simulink model "SWC_FDC_type"  (R2021b)
settings: Solver=FixedStepDiscrete  StartTime=0.0  StopTime=10.0  FixedStep=0.001  RelTol=1e-3
values from neighbouring files (symbols this model uses):
  C_TASK_5MS_S = (	C_TICK_TIME_S      	)    [vcu_local_hdr.m]
  DID_VCUKey = uint16(0x0202)    [vcu_local_hdr.m]
  DID_XWD = uint16(513)    [vcu_local_hdr.m]
  DIDLen_DKCKey = uint16(8)    [vcu_local_hdr.m]
  DIDLen_FoxPiBattSta = uint16(4)    [vcu_local_hdr.m]
  DIDLen_FoxPiBrakeSta = uint16(13)    [vcu_local_hdr.m]
  DIDLen_FoxPiButtonSta = uint16(2)    [vcu_local_hdr.m]
  DIDLen_FoxPiCtrlEnSw = uint16(1)    [vcu_local_hdr.m]
  DIDLen_FoxPiDrivingCtrl = uint16(21)    [vcu_local_hdr.m]
  DIDLen_FoxPiEPSSta = uint16(11)    [vcu_local_hdr.m]
  DIDLen_FoxPiLampCtrl = uint16(6)    [vcu_local_hdr.m]
  DIDLen_FoxPiLampSta = uint16(2)    [vcu_local_hdr.m]
  DIDLen_FoxPiMotionSta = uint16(13)    [vcu_local_hdr.m]
  DIDLen_FoxPiMotorSta = uint16(11)    [vcu_local_hdr.m]
  DIDLen_FoxPiPedalPos = uint16(3)    [vcu_local_hdr.m]
  DIDLen_FoxPiPTGUSSSw = uint16(1)    [vcu_local_hdr.m]
  DIDLen_FoxPiShifterAllow = uint16(3)    [vcu_local_hdr.m]
  DIDLen_FoxPiSwSta = uint16(2)    [vcu_local_hdr.m]
  DIDLen_FoxPiTPMSSta = uint16(13)    [vcu_local_hdr.m]
  DIDLen_FoxPiUSSDist = uint16(20)    [vcu_local_hdr.m]
  DIDLen_FoxPiUSSFaultSta = uint16(2)    [vcu_local_hdr.m]
  DIDLen_FoxPiWheelSpd = uint16(16)    [vcu_local_hdr.m]
  DIDNum_DKCKey = uint16(0x0202)    [vcu_local_hdr.m]
  DIDNum_FoxPiBattSta = uint16(0x100D)    [vcu_local_hdr.m]
  DIDNum_FoxPiBrakeSta = uint16(0x1003)    [vcu_local_hdr.m]
  DIDNum_FoxPiButtonSta = uint16(0x1006)    [vcu_local_hdr.m]
  DIDNum_FoxPiCtrlEnSw = uint16(0x1012)    [vcu_local_hdr.m]
  DIDNum_FoxPiDrivingCtrl = uint16(0x1001)    [vcu_local_hdr.m]
  DIDNum_FoxPiEPSSta = uint16(0x1005)    [vcu_local_hdr.m]
  DIDNum_FoxPiLampCtrl = uint16(0x100C)    [vcu_local_hdr.m]
  DIDNum_FoxPiLampSta = uint16(0x100B)    [vcu_local_hdr.m]
  DIDNum_FoxPiMotionSta = uint16(0x1002)    [vcu_local_hdr.m]
  DIDNum_FoxPiMotorSta = uint16(0x1010)    [vcu_local_hdr.m]
  DIDNum_FoxPiPedalPos = uint16(0x100F)    [vcu_local_hdr.m]
  DIDNum_FoxPiPTGUSSSw = uint16(0x1009)    [vcu_local_hdr.m]
  DIDNum_FoxPiShifterAllow = uint16(0x1011)    [vcu_local_hdr.m]
  DIDNum_FoxPiSwSta = uint16(0x100A)    [vcu_local_hdr.m]
  DIDNum_FoxPiTPMSSta = uint16(0x100E)    [vcu_local_hdr.m]
  DIDNum_FoxPiUSSDist = uint16(0x1007)    [vcu_local_hdr.m]
  DIDNum_FoxPiUSSFaultSta = uint16(0x1008)    [vcu_local_hdr.m]
  DIDNum_FoxPiWheelSpd = uint16(0x1004)    [vcu_local_hdr.m]
  DIDVCUKeyLength = uint16(8)    [vcu_local_hdr.m]
  DTC_10020B = Simulink.Parameter    [DTC_Constant_Definition.m]
  DTC_10020C = Simulink.Parameter    [DTC_Constant_Definition.m]
  DTC_10020D = Simulink.Parameter    [DTC_Constant_Definition.m]
  DTC_10020E = Simulink.Parameter    [DTC_Constant_Definition.m]
  DTC_100210 = Simulink.Parameter    [DTC_Constant_Definition.m]
  DTC_100211 = Simulink.Parameter    [DTC_Constant_Definition.m]
  DTC_100212 = Simulink.Parameter    [DTC_Constant_Definition.m]
  DTC_100213 = Simulink.Parameter    [DTC_Constant_Definition.m]
  DTC_100214 = Simulink.Parameter    [DTC_Constant_Definition.m]
  DTC_100215 = Simulink.Parameter    [DTC_Constant_Definition.m]
  DTC_100216 = Simulink.Parameter    [DTC_Constant_Definition.m]
  DTC_100217 = Simulink.Parameter    [DTC_Constant_Definition.m]
  DTC_100218 = Simulink.Parameter    [DTC_Constant_Definition.m]
  DTC_100219 = Simulink.Parameter    [DTC_Constant_Definition.m]
  DTC_10021A = Simulink.Parameter    [DTC_Constant_Definition.m]
  DTC_10021B = Simulink.Parameter    [DTC_Constant_Definition.m]
  DTC_10021C = Simulink.Parameter    [DTC_Constant_Definition.m]
  DTC_10021D = Simulink.Parameter    [DTC_Constant_Definition.m]
  DTC_10021E = Simulink.Parameter    [DTC_Constant_Definition.m]
  DTC_100220 = Simulink.Parameter    [DTC_Constant_Definition.m]
  DTC_100221 = Simulink.Parameter    [DTC_Constant_Definition.m]
  DTC_100223 = Simulink.Parameter    [DTC_Constant_Definition.m]
  DTC_100224 = Simulink.Parameter    [DTC_Constant_Definition.m]
  DTC_100225 = Simulink.Parameter    [DTC_Constant_Definition.m]
  DTC_100226 = Simulink.Parameter    [DTC_Constant_Definition.m]
  DTC_100227 = Simulink.Parameter    [DTC_Constant_Definition.m]
  DTC_100242 = Simulink.Parameter    [DTC_Constant_Definition.m]
  DTC_100243 = Simulink.Parameter    [DTC_Constant_Definition.m]
  DTC_100244 = Simulink.Parameter    [DTC_Constant_Definition.m]
  DTC_100247 = Simulink.Parameter    [DTC_Constant_Definition.m]
  DTC_100248 = Simulink.Parameter    [DTC_Constant_Definition.m]
  DTC_100249 = Simulink.Parameter    [DTC_Constant_Definition.m]
  DTC_100250 = Simulink.Parameter    [DTC_Constant_Definition.m]
  DTC_100251 = Simulink.Parameter    [DTC_Constant_Definition.m]
  DTC_100252 = Simulink.Parameter    [DTC_Constant_Definition.m]
  DTC_100A10 = Simulink.Parameter    [DTC_Constant_Definition.m]
  DTC_100A12 = Simulink.Parameter    [DTC_Constant_Definition.m]
  DTC_100A16 = Simulink.Parameter    [DTC_Constant_Definition.m]
  DTC_100A17 = Simulink.Parameter    [DTC_Constant_Definition.m]
  DTC_100A18 = Simulink.Parameter    [DTC_Constant_Definition.m]
  DTC_100A19 = Simulink.Parameter    [DTC_Constant_Definition.m]
  DTC_500B01 = Simulink.Parameter    [DTC_Constant_Definition.m]
  DTC_500B02 = Simulink.Parameter    [DTC_Constant_Definition.m]
  DTC_500B03 = Simulink.Parameter    [DTC_Constant_Definition.m]
  DTC_500B04 = Simulink.Parameter    [DTC_Constant_Definition.m]
  DTC_500B05 = Simulink.Parameter    [DTC_Constant_Definition.m]
  DTC_500B06 = Simulink.Parameter    [DTC_Constant_Definition.m]
  DTC_500B07 = Simulink.Parameter    [DTC_Constant_Definition.m]
  DTC_500B08 = Simulink.Parameter    [DTC_Constant_Definition.m]
  DTC_500B09 = Simulink.Parameter    [DTC_Constant_Definition.m]
  DTC_500B0A = Simulink.Parameter    [DTC_Constant_Definition.m]
  DTC_500B0B = Simulink.Parameter    [DTC_Constant_Definition.m]
  DTC_500B0C = Simulink.Parameter    [DTC_Constant_Definition.m]
  DTC_500B0D = Simulink.Parameter    [DTC_Constant_Definition.m]
  DTC_500B0E = Simulink.Parameter    [DTC_Constant_Definition.m]
  DTC_500B0F = Simulink.Parameter    [DTC_Constant_Definition.m]
  DTC_500B10 = Simulink.Parameter    [DTC_Constant_Definition.m]
  DTC_90021F = Simulink.Parameter    [DTC_Constant_Definition.m]
  DTC_90022F = Simulink.Parameter    [DTC_Constant_Definition.m]
  DTC_900253 = Simulink.Parameter    [DTC_Constant_Definition.m]
  DTC_900254 = Simulink.Parameter    [DTC_Constant_Definition.m]
  DTC_900301 = Simulink.Parameter    [DTC_Constant_Definition.m]
  DTC_900302 = Simulink.Parameter    [DTC_Constant_Definition.m]
  DTC_900303 = Simulink.Parameter    [DTC_Constant_Definition.m]
  DTC_900304 = Simulink.Parameter    [DTC_Constant_Definition.m]
  DTC_900305 = Simulink.Parameter    [DTC_Constant_Definition.m]
  DTC_900909 = Simulink.Parameter    [DTC_Constant_Definition.m]
  DTC_90090A = Simulink.Parameter    [DTC_Constant_Definition.m]
  DTC_90090B = Simulink.Parameter    [DTC_Constant_Definition.m]
  DTC_90090C = Simulink.Parameter    [DTC_Constant_Definition.m]
  DTC_90090D = Simulink.Parameter    [DTC_Constant_Definition.m]
  DTC_90090E = Simulink.Parameter    [DTC_Constant_Definition.m]
  DTC_90090F = Simulink.Parameter    [DTC_Constant_Definition.m]
  DTC_900910 = Simulink.Parameter    [DTC_Constant_Definition.m]
  DTC_900911 = Simulink.Parameter    [DTC_Constant_Definition.m]
  DTC_900912 = Simulink.Parameter    [DTC_Constant_Definition.m]
  DTC_900913 = Simulink.Parameter    [DTC_Constant_Definition.m]
  DTC_900914 = Simulink.Parameter    [DTC_Constant_Definition.m]
  ... (+54 more)
undefined symbols (not defined in the file or in its folder): f32_ApsOutVehSpdSig, KHAL_CANBusOffDebounce_cnt, KHAL_CANBusOffDebounce_s, KHAL_DKCDecryptEnable_flg_ovrdflg, KHAL_DKCDecryptEnable_flg_ovrdval, KHAL_RandomNumberY1_enum, KHAL_RandomNumberY2_enum, KHAL_RandomNumberY_ovrdflg, KHAL_TPMSRESBUTT_flg_ovrdflg, KHAL_TPMSRESBUTT_flg_ovrdval, KINP_ReadVinCode_flg, P_boolean, R_DIDWriteCDD_CSOP_DIDSet_DKCKey, R_DIDWriteCDD_CSOP_DIDSet_FoxPiBattSta, R_DIDWriteCDD_CSOP_DIDSet_FoxPiBrakeSta, R_DIDWriteCDD_CSOP_DIDSet_FoxPiButtonSta, R_DIDWriteCDD_CSOP_DIDSet_FoxPiCtrlEnSw, R_DIDWriteCDD_CSOP_DIDSet_FoxPiDrivingCtrl, R_DIDWriteCDD_CSOP_DIDSet_FoxPiEPSSta, R_DIDWriteCDD_CSOP_DIDSet_FoxPiLampCtrl, R_DIDWriteCDD_CSOP_DIDSet_FoxPiLampSta, R_DIDWriteCDD_CSOP_DIDSet_FoxPiMotionSta, R_DIDWriteCDD_CSOP_DIDSet_FoxPiMotorSta, R_DIDWriteCDD_CSOP_DIDSet_FoxPiPedalPos, R_DIDWriteCDD_CSOP_DIDSet_FoxPiPTGUSSSw, R_DIDWriteCDD_CSOP_DIDSet_FoxPiShifterAllow, R_DIDWriteCDD_CSOP_DIDSet_FoxPiSwSta, R_DIDWriteCDD_CSOP_DIDSet_FoxPiTPMSSta, R_DIDWriteCDD_CSOP_DIDSet_FoxPiUSSDist, R_DIDWriteCDD_CSOP_DIDSet_FoxPiUSSFaultSta, R_DIDWriteCDD_CSOP_DIDSet_FoxPiWheelSpd, R_E2E_CAN3_VCU1_CSOP_Write_CAN3_VCU1, R_E2E_CAN3_VCU1_toNIDEC_CSOP_Write_CAN3_VCU1_toNIDEC, R_E2E_CAN4_VCU1_CSOP_Write_CAN4_VCU1, R_FDCCDD_Inner_CSOP_FDC_AppCallSleep, R_HALIN_IMU_CSOP_IMUSetSta, R_HALINCDD_CSOP_PAS_Handler, R_HALINCDD_CSOP_ResetPedalZeroPosDone, R_HALINCDD_CSOP_TPMSSensorIDRegSetResults, R_HALINCDD_CSOP_UDS_Main, R_HALOUT_APS_CSOP_ApsOutput, R_HALOUTCDD_CSOP_AppNmStateReq, R_HALOUTCDD_CSOP_IVIReset, R_HALOUTCDD_CSOP_SetAcoreRebootCmdACK, R_HALOUTCDD_CSOP_SetSysPwrStat ... (+80)
libraries: FVT_lib x447, simulink x289, hcu_lib x19, hdlsllib x9, app x1, halin x1, halout x1, matrix_library x1, inp x1, outp x1
(part 13 of 15)

== system SWC_FDC_type/run_SWC_FDC_RxTx_5ms_sys/Halin_CDD/Halin_TPMS/Subsystem ==
  note: Custom State Judgement
  note: Data Output
  note: Data Valid Judge
  TPMS_DataIn_flg : Inport
  TPMS_RawData : Inport  Port=2
  Add : Sum  Inputs=++++
  Bit Shift : hdlsllib/Logic and Bit Operations/Bit Shift  mode=Shift Left Logical  N=24
  Bit Shift1 : hdlsllib/Logic and Bit Operations/Bit Shift  mode=Shift Left Logical  N=16
  Bit Shift3 : hdlsllib/Logic and Bit Operations/Bit Shift  mode=Shift Left Logical  N=8
  Bitwise NOT : simulink/Logic and Bit Operations/Bitwise Operator  logicop=NOT  UseBitMask=off  BitMask=bin2dec('11011001')  BitMaskRealWorld=Stored Integer
  CRC8_Caculation : Subsystem
  Constant1 : Constant  Value=ENUM_TPMSSTA_TRIGGER
  Constant{4,7,9..10} (4 alike) : Constant  Value=TRUE
  Constant{5..6,8,11} (4 alike) : Constant  Value=FALSE
  Constant2 : Constant  Value=ENUM_TPMSSTA_LOWBATTERY
  Constant3 : Constant  Value=ENUM_TPMSSTA_FAT
  Data Type Conversion : DataTypeConversion  OutDataTypeStr=uint32
  Data Type Conversion1 : DataTypeConversion  OutDataTypeStr=uint8
  Data Type Conversion2 : DataTypeConversion  OutDataTypeStr=uint8
  Data Type Conversion3 : DataTypeConversion  OutDataTypeStr=uint32
  Data Type Conversion4 : DataTypeConversion  OutDataTypeStr=uint32
  Demux : Demux  Outputs=9
  Demux1 : Demux  Outputs=10
  Equal{,1..4} (5 alike) : RelationalOperator  Operator===  OutDataTypeStr=boolean  RndMeth=Simplest
  Logical Operator : Logic  Inputs=3  AllPortsSameDT=off  OutDataTypeStr=boolean
  Mux : Mux  Inputs=10
  Mux1 : Mux  Inputs=8
  Switch{,1..4} (5 alike) : Switch  Criteria=u2 ~= 0
  Unit Delay : UnitDelay  SampleTime=-1  HasFrameUpgradeWarning=on
  VHAL_TPMSDataIn_flg : Outport
  VHAL_TPMSID_raw : Outport  Port=2
  VHAL_TPMSPressure_raw : Outport  Port=3
  VHAL_TPMSTemp_raw : Outport  Port=4
  VHAL_TPMSSta_enum : Outport  Port=5
  VHAL_TPMSPressureMi_raw : Outport  Port=6
  VHAL_TPMSCRC_crc : Outport  Port=7
  VHAL_TPMSCRCCalc_crc : Outport  Port=8
  VHAL_TPMSFAT_flg : Outport  Port=9
  VHAL_TPMSBattLow_flg : Outport  Port=10
  VHAL_TPMSTrigger_flg : Outport  Port=11
  wires:
  TPMS_DataIn_flg/1 -> Data Type Conversion2/1
  [TPMSData] -> Demux/1
  Bit Shift/1 -> Add/1
  Bit Shift1/1 -> Add/2
  Bit Shift3/1 -> Add/3
  Add/1 -> VHAL_TPMSID_raw/1
  Demux/5 -> [Pressure]  "Pressure"
  Demux/7 -> [Status]  "Sta"
  Demux/8 -> [PressureMirror]  "PressureMirror"
  Demux/9 -> [CRC]  "CRC"
  Demux/1 -> [ID4]  "ID4"
  Demux/2 -> [ID3]  "ID3"
  Demux/3 -> [ID2]  "ID2"
  Demux/4 -> [ID1]  "ID1"
  Demux/6 -> [Temp]  "Temp"
  [Pressure] -> Bitwise NOT/1
  Bitwise NOT/1 -> Equal/1
  [PressureMirror] -> Equal/2
  [ID4] -> Mux1/1
  [ID3] -> Mux1/2
  [ID2] -> Mux1/3
  [ID1] -> Mux1/4
  [Pressure] -> Mux1/5
  [Temp] -> Mux1/6
  [Status] -> Mux1/7
  [PressureMirror] -> Mux1/8
  Mux1/1 -> CRC8_Caculation/1(MsgData)
  [CRC] -> Equal1/2
  Equal1/1 -> Logical Operator/1
  Equal/1 -> Logical Operator/2
  Logical Operator/1 -> [DataValid_flg]
  [DataValid_flg] -> Switch/2
  Mux/1 -> Switch/1
  Switch/1 -> Unit Delay/1, Demux1/1
  Unit Delay/1 -> Switch/3
  Data Type Conversion1/1 -> [TPMSData]
  Data Type Conversion2/1 -> [Data_in]
  CRC8_Caculation/1(CRCout) -> [CRC_Calc], Equal1/1  "CRC_Calc"
  Switch1/1 -> VHAL_TPMSFAT_flg/1
  [VHAL_TPMSSta_enum] -> Equal2/1
  Constant3/1 -> Equal2/2
  Equal2/1 -> Switch1/2
  Constant4/1 -> Switch1/1
  Constant5/1 -> Switch1/3
  Constant8/1 -> Switch2/3
  [VHAL_TPMSSta_enum] -> Equal3/1
  Constant7/1 -> Switch2/1
  Switch2/1 -> VHAL_TPMSBattLow_flg/1
  Equal3/1 -> Switch2/2
  Constant2/1 -> Equal3/2
  [Data_in] -> Logical Operator/3
  [DataValid_flg] -> Switch3/2
  Switch3/1 -> VHAL_TPMSDataIn_flg/1
  Constant6/1 -> Switch3/3
  Constant9/1 -> Switch3/1
  [ID4] -> Mux/1
  [ID3] -> Mux/2
  [ID2] -> Mux/3
  [ID1] -> Mux/4
  [Pressure] -> Mux/5
  [Temp] -> Mux/6
  [Status] -> Mux/7
  [PressureMirror] -> Mux/8
  [CRC] -> Mux/9
  [CRC_Calc] -> Mux/10
  Demux1/10 -> VHAL_TPMSCRCCalc_crc/1
  Demux1/9 -> VHAL_TPMSCRC_crc/1
  Demux1/8 -> VHAL_TPMSPressureMi_raw/1
  Demux1/7 -> [VHAL_TPMSSta_enum], VHAL_TPMSSta_enum/1
  Demux1/6 -> VHAL_TPMSTemp_raw/1
  Demux1/5 -> VHAL_TPMSPressure_raw/1
  Demux1/1 -> Data Type Conversion/1
  Demux1/2 -> Data Type Conversion3/1
  Demux1/3 -> Data Type Conversion4/1
  Data Type Conversion/1 -> Bit Shift/1
  Data Type Conversion3/1 -> Bit Shift1/1
  Data Type Conversion4/1 -> Bit Shift3/1
  Demux1/4 -> Add/4
  TPMS_RawData/1 -> Data Type Conversion1/1
  [VHAL_TPMSSta_enum] -> Equal4/1
  Constant1/1 -> Equal4/2
  Equal4/1 -> Switch4/2
  Constant10/1 -> Switch4/1
  Constant11/1 -> Switch4/3
  Switch4/1 -> VHAL_TPMSTrigger_flg/1

== system SWC_FDC_type/run_SWC_FDC_RxTx_5ms_sys/OUTP_AFTER/DID_list/pct2raw1 ==
  EAPS1_pct : Inport
  EAPS2_pct : Inport  Port=2
  Bitwise AND1 : simulink/Logic and Bit Operations/Bitwise Operator  logicop=AND  UseBitMask=on  BitMask=0xF  BitMaskRealWorld=Stored Integer
  Bitwise AND2 : simulink/Logic and Bit Operations/Bitwise Operator  logicop=AND  UseBitMask=on  BitMask=0xFF0  BitMaskRealWorld=Stored Integer
  Bitwise AND3 : simulink/Logic and Bit Operations/Bitwise Operator  logicop=AND  UseBitMask=on  BitMask=0xFF  BitMaskRealWorld=Stored Integer
  Bitwise AND4 : simulink/Logic and Bit Operations/Bitwise Operator  logicop=AND  UseBitMask=on  BitMask=0xF00  BitMaskRealWorld=Stored Integer
  Bitwise AND5 : simulink/Logic and Bit Operations/Bitwise Operator  logicop=OR  UseBitMask=off  NumInputPorts=2  BitMask=0xFF  BitMaskRealWorld=Stored Integer
  Data Type Conversion1 : DataTypeConversion  OutDataTypeStr=uint8
  Data Type Conversion2 : DataTypeConversion  OutDataTypeStr=uint16
  Data Type Conversion3 : DataTypeConversion  OutDataTypeStr=uint8
  Data Type Conversion4 : DataTypeConversion  OutDataTypeStr=uint16
  Data Type Conversion5 : DataTypeConversion  OutDataTypeStr=uint8
  Gain : Gain  Gain=1/20
  Gain1 : Gain  Gain=1/40
  Mux2 : Mux  Inputs=3
  Shift Arithmetic1 : ArithShift  BitShiftNumber=8  BitShiftDirection=Right
  Shift Arithmetic2 : ArithShift  BitShiftNumber=4  BitShiftDirection=Left
  Shift Arithmetic39 : ArithShift  BitShiftNumber=4  BitShiftDirection=Right
  convert_out1 : FVT_lib/hal/convert_out  gain=0.001  offset=0
  convert_out4 : FVT_lib/hal/convert_out  gain=0.001  offset=0
  PedalZP_raw8 : Outport
  wires:
  Data Type Conversion1/1 -> Mux2/2
  Bitwise AND5/1 -> Data Type Conversion1/1
  Shift Arithmetic1/1 -> Bitwise AND5/2
  Shift Arithmetic2/1 -> Bitwise AND5/1
  Gain1/1 -> convert_out1/1
  Gain/1 -> convert_out4/1
  EAPS1_pct/1 -> Gain/1
  convert_out4/1 -> Data Type Conversion2/1
  convert_out1/1 -> Data Type Conversion4/1
  EAPS2_pct/1 -> Gain1/1
  Bitwise AND3/1 -> Data Type Conversion3/1
  Bitwise AND4/1 -> Shift Arithmetic1/1
  Data Type Conversion4/1 -> Bitwise AND3/1, Bitwise AND4/1
  Data Type Conversion3/1 -> Mux2/3
  Data Type Conversion5/1 -> Mux2/1
  Data Type Conversion2/1 -> Bitwise AND2/1, Bitwise AND1/1
  Bitwise AND2/1 -> Shift Arithmetic39/1
  Shift Arithmetic39/1 -> Data Type Conversion5/1
  Mux2/1 -> PedalZP_raw8/1
  Bitwise AND1/1 -> Shift Arithmetic2/1

== system SWC_FDC_type/run_SWC_FDC_RxTx_5ms_sys/OUTP_AFTER/DID_list/pct2raw8 ==
  EAPS1_pct : Inport
  EAPS2_pct : Inport  Port=2
  Bitwise AND1 : simulink/Logic and Bit Operations/Bitwise Operator  logicop=AND  UseBitMask=on  BitMask=0xF  BitMaskRealWorld=Stored Integer
  Bitwise AND2 : simulink/Logic and Bit Operations/Bitwise Operator  logicop=AND  UseBitMask=on  BitMask=0xFF0  BitMaskRealWorld=Stored Integer
  Bitwise AND3 : simulink/Logic and Bit Operations/Bitwise Operator  logicop=AND  UseBitMask=on  BitMask=0xFF  BitMaskRealWorld=Stored Integer
  Bitwise AND4 : simulink/Logic and Bit Operations/Bitwise Operator  logicop=AND  UseBitMask=on  BitMask=0xF00  BitMaskRealWorld=Stored Integer
  Bitwise AND5 : simulink/Logic and Bit Operations/Bitwise Operator  logicop=OR  UseBitMask=off  NumInputPorts=2  BitMask=0xFF  BitMaskRealWorld=Stored Integer
  Data Type Conversion1 : DataTypeConversion  OutDataTypeStr=uint8
  Data Type Conversion2 : DataTypeConversion  OutDataTypeStr=uint16
  Data Type Conversion3 : DataTypeConversion  OutDataTypeStr=uint8
  Data Type Conversion4 : DataTypeConversion  OutDataTypeStr=uint16
  Data Type Conversion5 : DataTypeConversion  OutDataTypeStr=uint8
  Gain : Gain  Gain=1/20
  Gain1 : Gain  Gain=1/40
  Mux2 : Mux  Inputs=3
  Shift Arithmetic1 : ArithShift  BitShiftNumber=8  BitShiftDirection=Right
  Shift Arithmetic2 : ArithShift  BitShiftNumber=4  BitShiftDirection=Left
  Shift Arithmetic39 : ArithShift  BitShiftNumber=4  BitShiftDirection=Right
  convert_out1 : FVT_lib/hal/convert_out  gain=0.001  offset=0
  convert_out4 : FVT_lib/hal/convert_out  gain=0.001  offset=0
  PedalZP_raw8 : Outport
  wires:
  Bitwise AND1/1 -> Shift Arithmetic2/1
  Mux2/1 -> PedalZP_raw8/1
  Shift Arithmetic39/1 -> Data Type Conversion5/1
  Bitwise AND2/1 -> Shift Arithmetic39/1
  Data Type Conversion2/1 -> Bitwise AND1/1, Bitwise AND2/1
  Data Type Conversion5/1 -> Mux2/1
  Data Type Conversion3/1 -> Mux2/3
  Data Type Conversion4/1 -> Bitwise AND4/1, Bitwise AND3/1
  Bitwise AND4/1 -> Shift Arithmetic1/1
  Bitwise AND3/1 -> Data Type Conversion3/1
  EAPS2_pct/1 -> Gain1/1
  convert_out1/1 -> Data Type Conversion4/1
  convert_out4/1 -> Data Type Conversion2/1
  EAPS1_pct/1 -> Gain/1
  Gain/1 -> convert_out4/1
  Gain1/1 -> convert_out1/1
  Shift Arithmetic2/1 -> Bitwise AND5/1
  Shift Arithmetic1/1 -> Bitwise AND5/2
  Bitwise AND5/1 -> Data Type Conversion1/1
  Data Type Conversion1/1 -> Mux2/2

== system SWC_FDC_type/run_SWC_FDC_RxTx_5ms_sys/OUTP_AFTER/DID_list/uint32Touint8Array ==
  In1 : Inport
  Bitwise AND1 : simulink/Logic and Bit Operations/Bitwise Operator  logicop=AND  UseBitMask=on  BitMask=bin2dec('00000000000000000000000011111111')  BitMaskRealWorld=Stored Integer
  Bitwise AND2 : simulink/Logic and Bit Operations/Bitwise Operator  logicop=AND  UseBitMask=on  BitMask=bin2dec('00000000000000001111111100000000')  BitMaskRealWorld=Stored Integer
  Bitwise AND3 : simulink/Logic and Bit Operations/Bitwise Operator  logicop=AND  UseBitMask=on  BitMask=bin2dec('00000000111111110000000000000000')  BitMaskRealWorld=Stored Integer
  Bitwise AND4 : simulink/Logic and Bit Operations/Bitwise Operator  logicop=AND  UseBitMask=on  BitMask=bin2dec('11111111000000000000000000000000')  BitMaskRealWorld=Stored Integer
  Data Type Conversion{1,3..5} (4 alike) : DataTypeConversion  OutDataTypeStr=uint8
  Data Type Conversion2 : DataTypeConversion  OutDataTypeStr=uint32
  Mux2 : Mux
  Shift Arithmetic39 : ArithShift  BitShiftNumber=8  BitShiftDirection=Right
  Shift Arithmetic40 : ArithShift  BitShiftNumber=16  BitShiftDirection=Right
  Shift Arithmetic41 : ArithShift  BitShiftNumber=24  BitShiftDirection=Right
  Out1 : Outport
  wires:
  Bitwise AND4/1 -> Shift Arithmetic41/1
  Bitwise AND1/1 -> Data Type Conversion1/1
  Shift Arithmetic40/1 -> Data Type Conversion4/1
  Shift Arithmetic41/1 -> Data Type Conversion3/1
  Mux2/1 -> Out1/1
  In1/1 -> Data Type Conversion2/1
  Bitwise AND3/1 -> Shift Arithmetic40/1
  Shift Arithmetic39/1 -> Data Type Conversion5/1
  Data Type Conversion3/1 -> Mux2/1
  Bitwise AND2/1 -> Shift Arithmetic39/1
  Data Type Conversion2/1 -> Bitwise AND4/1, Bitwise AND3/1, Bitwise AND1/1, Bitwise AND2/1
  Data Type Conversion5/1 -> Mux2/3
  Data Type Conversion4/1 -> Mux2/2
  Data Type Conversion1/1 -> Mux2/4

== system SWC_FDC_type/run_SWC_FDC_RxTx_5ms_sys/OUTP_AFTER/DID_list/uint32Touint8Array1 ==
  In1 : Inport
  Bitwise AND1 : simulink/Logic and Bit Operations/Bitwise Operator  logicop=AND  UseBitMask=on  BitMask=bin2dec('00000000000000000000000011111111')  BitMaskRealWorld=Stored Integer
  Bitwise AND2 : simulink/Logic and Bit Operations/Bitwise Operator  logicop=AND  UseBitMask=on  BitMask=bin2dec('00000000000000001111111100000000')  BitMaskRealWorld=Stored Integer
  Bitwise AND3 : simulink/Logic and Bit Operations/Bitwise Operator  logicop=AND  UseBitMask=on  BitMask=bin2dec('00000000111111110000000000000000')  BitMaskRealWorld=Stored Integer
  Bitwise AND4 : simulink/Logic and Bit Operations/Bitwise Operator  logicop=AND  UseBitMask=on  BitMask=bin2dec('11111111000000000000000000000000')  BitMaskRealWorld=Stored Integer
  Data Type Conversion{1,3..5} (4 alike) : DataTypeConversion  OutDataTypeStr=uint8
  Data Type Conversion2 : DataTypeConversion  OutDataTypeStr=uint32
  Mux2 : Mux
  Shift Arithmetic39 : ArithShift  BitShiftNumber=8  BitShiftDirection=Right
  Shift Arithmetic40 : ArithShift  BitShiftNumber=16  BitShiftDirection=Right
  Shift Arithmetic41 : ArithShift  BitShiftNumber=24  BitShiftDirection=Right
  Out1 : Outport
  wires:
  Data Type Conversion1/1 -> Mux2/4
  Data Type Conversion4/1 -> Mux2/2
  Data Type Conversion5/1 -> Mux2/3
  Data Type Conversion2/1 -> Bitwise AND2/1, Bitwise AND1/1, Bitwise AND3/1, Bitwise AND4/1
  Bitwise AND2/1 -> Shift Arithmetic39/1
  Data Type Conversion3/1 -> Mux2/1
  Shift Arithmetic39/1 -> Data Type Conversion5/1
  Bitwise AND3/1 -> Shift Arithmetic40/1
  In1/1 -> Data Type Conversion2/1
  Mux2/1 -> Out1/1
  Shift Arithmetic41/1 -> Data Type Conversion3/1
  Shift Arithmetic40/1 -> Data Type Conversion4/1
  Bitwise AND1/1 -> Data Type Conversion1/1
  Bitwise AND4/1 -> Shift Arithmetic41/1

== system SWC_FDC_type/run_SWC_FDC_RxTx_5ms_sys/OUTP_AFTER/DID_list/uint32Touint8Array2 ==
  In1 : Inport
  Bitwise AND1 : simulink/Logic and Bit Operations/Bitwise Operator  logicop=AND  UseBitMask=on  BitMask=bin2dec('00000000000000000000000011111111')  BitMaskRealWorld=Stored Integer
  Bitwise AND2 : simulink/Logic and Bit Operations/Bitwise Operator  logicop=AND  UseBitMask=on  BitMask=bin2dec('00000000000000001111111100000000')  BitMaskRealWorld=Stored Integer
  Bitwise AND3 : simulink/Logic and Bit Operations/Bitwise Operator  logicop=AND  UseBitMask=on  BitMask=bin2dec('00000000111111110000000000000000')  BitMaskRealWorld=Stored Integer
  Bitwise AND4 : simulink/Logic and Bit Operations/Bitwise Operator  logicop=AND  UseBitMask=on  BitMask=bin2dec('11111111000000000000000000000000')  BitMaskRealWorld=Stored Integer
  Data Type Conversion{1,3..5} (4 alike) : DataTypeConversion  OutDataTypeStr=uint8
  Data Type Conversion2 : DataTypeConversion  OutDataTypeStr=uint32
  Mux2 : Mux
  Shift Arithmetic39 : ArithShift  BitShiftNumber=8  BitShiftDirection=Right
  Shift Arithmetic40 : ArithShift  BitShiftNumber=16  BitShiftDirection=Right
  Shift Arithmetic41 : ArithShift  BitShiftNumber=24  BitShiftDirection=Right
  Out1 : Outport
  wires:
  Bitwise AND4/1 -> Shift Arithmetic41/1
  Bitwise AND1/1 -> Data Type Conversion1/1
  Shift Arithmetic40/1 -> Data Type Conversion4/1
  Shift Arithmetic41/1 -> Data Type Conversion3/1
  Mux2/1 -> Out1/1
  In1/1 -> Data Type Conversion2/1
  Bitwise AND3/1 -> Shift Arithmetic40/1
  Shift Arithmetic39/1 -> Data Type Conversion5/1
  Data Type Conversion3/1 -> Mux2/1
  Bitwise AND2/1 -> Shift Arithmetic39/1
  Data Type Conversion2/1 -> Bitwise AND4/1, Bitwise AND3/1, Bitwise AND1/1, Bitwise AND2/1
  Data Type Conversion5/1 -> Mux2/3
  Data Type Conversion4/1 -> Mux2/2
  Data Type Conversion1/1 -> Mux2/4

== system SWC_FDC_type/run_SWC_FDC_RxTx_5ms_sys/OUTP_AFTER/DID_list/uint32Touint8Array3 ==
  In1 : Inport
  Bitwise AND1 : simulink/Logic and Bit Operations/Bitwise Operator  logicop=AND  UseBitMask=on  BitMask=bin2dec('00000000000000000000000011111111')  BitMaskRealWorld=Stored Integer
  Bitwise AND2 : simulink/Logic and Bit Operations/Bitwise Operator  logicop=AND  UseBitMask=on  BitMask=bin2dec('00000000000000001111111100000000')  BitMaskRealWorld=Stored Integer
  Bitwise AND3 : simulink/Logic and Bit Operations/Bitwise Operator  logicop=AND  UseBitMask=on  BitMask=bin2dec('00000000111111110000000000000000')  BitMaskRealWorld=Stored Integer
  Bitwise AND4 : simulink/Logic and Bit Operations/Bitwise Operator  logicop=AND  UseBitMask=on  BitMask=bin2dec('11111111000000000000000000000000')  BitMaskRealWorld=Stored Integer
  Data Type Conversion{1,3..5} (4 alike) : DataTypeConversion  OutDataTypeStr=uint8
  Data Type Conversion2 : DataTypeConversion  OutDataTypeStr=uint32
  Mux2 : Mux
  Shift Arithmetic39 : ArithShift  BitShiftNumber=8  BitShiftDirection=Right
  Shift Arithmetic40 : ArithShift  BitShiftNumber=16  BitShiftDirection=Right
  Shift Arithmetic41 : ArithShift  BitShiftNumber=24  BitShiftDirection=Right
  Out1 : Outport
  wires:
  Data Type Conversion1/1 -> Mux2/4
  Data Type Conversion4/1 -> Mux2/2
  Data Type Conversion5/1 -> Mux2/3
  Data Type Conversion2/1 -> Bitwise AND2/1, Bitwise AND1/1, Bitwise AND3/1, Bitwise AND4/1
  Bitwise AND2/1 -> Shift Arithmetic39/1
  Data Type Conversion3/1 -> Mux2/1
  Shift Arithmetic39/1 -> Data Type Conversion5/1
  Bitwise AND3/1 -> Shift Arithmetic40/1
  In1/1 -> Data Type Conversion2/1
  Mux2/1 -> Out1/1
  Shift Arithmetic41/1 -> Data Type Conversion3/1
  Shift Arithmetic40/1 -> Data Type Conversion4/1
  Bitwise AND1/1 -> Data Type Conversion1/1
  Bitwise AND4/1 -> Shift Arithmetic41/1
